simulink model "SMA_Model_with_Inverter_2021a"  (R2021a)
settings: Solver=ode45  StartTime=0.0  StopTime=300.0  FixedStep=1e-4  RelTol=1e-3
values from neighbouring files (symbols this model uses):
  a0 = 8.7e-7    (= 8.7e-07)    [Model_Parameters.m]
  a1 = 4.8e-8    (= 4.8e-08)    [Model_Parameters.m]
  a2 = -7.8e-9    (= -7.8e-09)    [Model_Parameters.m]
  a3 = 7e-10    [Model_Parameters.m]
  a4 = 3.7e-11    [Model_Parameters.m]
  c_heat = 837.36    [Model_Parameters.m]
  Capacitance = 10e-3    (= 0.01)    [Model_Parameters.m]
  CarrierFrequency = 1e-3    (= 0.001)    [Model_Parameters.m]
  Delta = 4.425e-2    (= 0.04425)    [Model_Parameters.m]
  do = 5e-4    (= 0.0005)    [Model_Parameters.m]
  Ea = 79    [Model_Parameters.m]
  Em = 34    [Model_Parameters.m]
  h = 70    [Model_Parameters.m]
  Initial_Rm = 1    [Model_Parameters.m]
  Initial_temperature = T_amb    (= 20)    [Model_Parameters.m]
  k = 58.19    [Model_Parameters.m]
  k1 = 0.0204    [Model_Parameters.m]
  k2 = 0.01293    [Model_Parameters.m]
  L = 0    [Model_Parameters.m]
  lo = 0.96    [Model_Parameters.m]
  m3 = 70    [Model_Parameters.m]
  mu_minus = 57    [Model_Parameters.m]
  mu_plus = 72    [Model_Parameters.m]
  n3 = 3    [Model_Parameters.m]
  ni_minus = 1    [Model_Parameters.m]
  ni_plus = 1    [Model_Parameters.m]
  p1 = 9.2e-7    (= 9.2e-07)    [Model_Parameters.m]
  p2 = 8.4e-7    (= 8.4e-07)    [Model_Parameters.m]
  p3 = 0.2499    [Model_Parameters.m]
  q1 = 3.4e-8    (= 3.4e-08)    [Model_Parameters.m]
  q2 = 5.7e-10    [Model_Parameters.m]
  R = 4.3    [Model_Parameters.m]
  rho = 6450    [Model_Parameters.m]
  sigma_minus = 1.6    [Model_Parameters.m]
  sigma_plus = 1.5    [Model_Parameters.m]
  Slider_Friction = 0.11    [Model_Parameters.m]
  SupplyInternalInductance = 0.4e-3    (= 0.0004)    [Model_Parameters.m]
  SupplyInternalResistance = 0.4    [Model_Parameters.m]
  SupplyVoltage = 80    [Model_Parameters.m]
  T_amb = 20    [Model_Parameters.m]
undefined symbols (not defined in the file or in its folder): CapacitanceResistance
libraries: fl_lib x7, spsVoltageMeasurementLib x6, spsDiodeLib x5, spsIdealSwitchLib x5, spsCurrentMeasurementLib x4, nesl_utility x4, spsSeriesRLCBranchLib x4, simulink x2, spsDCVoltageSourceLib x1, spspowerguiLib x1
settings Model: Creator=barag  LastModifiedBy=barag
settings SolverCC: ZeroCrossAlgorithm=Adaptive
settings DebuggingCC: MaskedZcDiagnostic=none  IgnoredZcDiagnostic=none

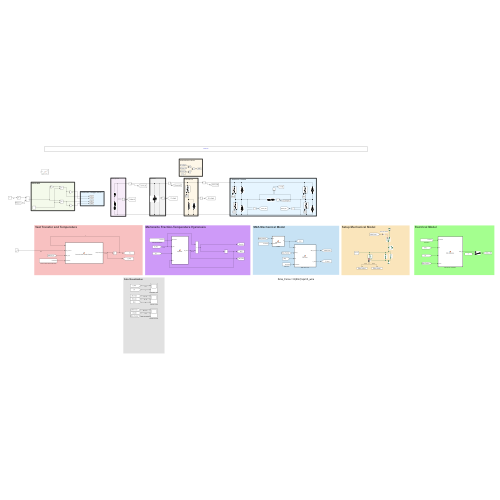
[thumbnail: Simulink's stored preview of the top-level diagram]
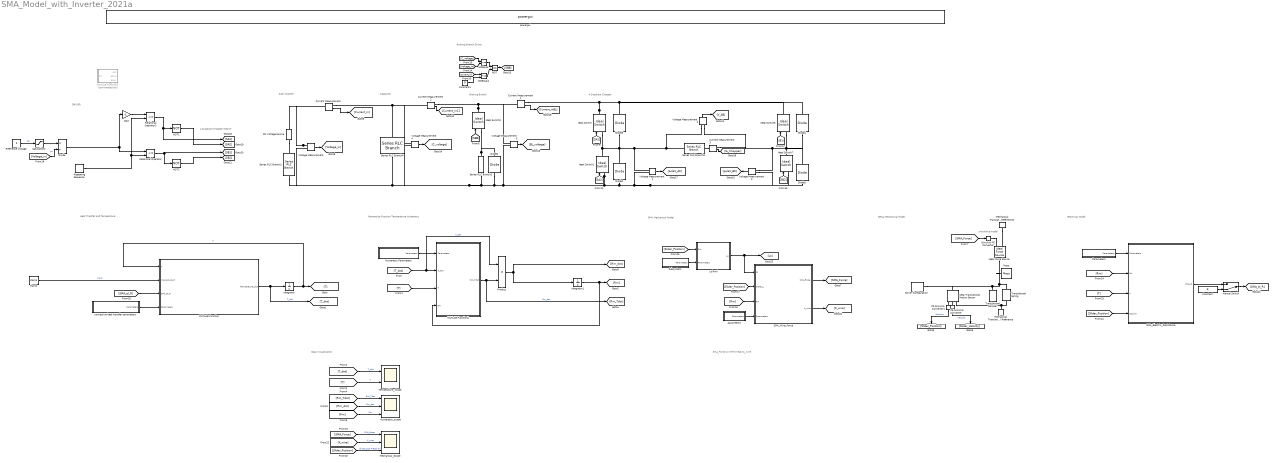
== system SMA_Model_with_Inverter_2021a ==
  note: Electrical Model
  note: Sma_Force = K(Rm)*eps*A_wire
  note: SMA Mechanical Model
  note: Setup Mechanical Model
  note: sma force model
  note: Data Visualization
  note: Martensite Fraction-Temperature Hysteresis
  note: Heat Transfer and Temperature
  note: Braking Branch
  note: Capacitor
  note: 4 Quadrant Chopper
  note: Braking Branch Driver
  note: Suply System
  note: DRIVER
  note: 4 Quadrant Chopper IN/OUT
  Constant : Constant  Value=R
  Constant1 : Constant  Value=0
  Current Measurement{,1..3} (4 alike) : spsCurrentMeasurementLib/Current Measurement  PhasorSimulation=off  OutputType=Complex  PSBequivalent=0
  DC Voltage Source : spsDCVoltageSourceLib/DC Voltage Source  Amplitude=SupplyVoltage  Measurements=None
  Diode{1..5} (5 alike) : spsDiodeLib/Diode  Ron=DiodeResistance  Lon=0  Vf=DiodeVfm  IC=0  UseSnubber=0  Rs=DiodeResistance  Cs=inf  Measurements=off
  Divide : Product  Inputs=*/
  Gain : Gain  Gain=-1
  Hysteresis Parameters : Subsystem
  Hysteresis_scope : Scope  NumInputPorts=3
  Ideal Force Source : fl_lib/Mechanical/Mechanical Sources/Ideal Force Source
  Ideal Switch{,1..2,6..7} (5 alike) : spsIdealSwitchLib/Ideal Switch  Ron=MosfetResistance  Lon=0  IC=0  Rs=DiodeResistance  Cs=inf  Measurements=off
  Ideal Translational Motion Sensor : fl_lib/Mechanical/Mechanical Sensors/Ideal Translational Motion Sensor  offset=4 cm
  Integrator : Integrator  InitialCondition=Initial_temperature
  Integrator1 : Integrator  InitialCondition=Initial_Rm
  Lo(Rm) : MATLAB Function  TreatAsAtomicUnit=on
  MATLAB Function : MATLAB Function  TreatAsAtomicUnit=on
  MATLAB Function1 : MATLAB Function  Commented=on  TreatAsAtomicUnit=on
  MATLAB Function2 : MATLAB Function  TreatAsAtomicUnit=on
  Manual Switch : ManualSwitch  CurrentSetting=0
  Mass : fl_lib/Mechanical/Translational Elements/Mass  mass=Slider_Mass kg  num_ports=foundation.enum.numPorts2.one  v_specify=off  v_priority=High  v=0 m/s  v_nominal_specify=off  v_nominal_unit=m/s  v_nominal_value=1  f_specify=off  f_priority=None  f=0 N  f_nominal_specify=off  f_nominal_unit=N  f_nominal_value=1
  Mechanical Translational Reference : fl_lib/Mechanical/Translational Elements/Mechanical Translational Reference
  Mechanical Translational Reference1 : fl_lib/Mechanical/Translational Elements/Mechanical Translational Reference
  Mechanical_Scope : Scope  NumInputPorts=3
  NOT : Logic  IconShape=distinctive  AllPortsSameDT=off  OutDataTypeStr=boolean
  NOT1 : Logic  Operator=NOT  IconShape=distinctive  AllPortsSameDT=off  OutDataTypeStr=boolean
  NOT2 : Logic  Operator=NOT  IconShape=distinctive  AllPortsSameDT=off  OutDataTypeStr=boolean
  NotEqual : RelationalOperator  Operator=~=  OutDataTypeStr=boolean  RndMeth=Simplest
  NotEqual1 : RelationalOperator  Operator=<=  OutDataTypeStr=boolean  RndMeth=Simplest
  PS-Simulink Converter : nesl_utility/PS-Simulink Converter  PhysicalDomain=network_engine_domain  SubClassName=ps_output  LeftPortType=input  RightPortType=output  PseudoPeriodic=off  Frequencies=[]  Unit=inherit  AffineConversion=off
      settings: SourceProductBaseCode=PW,SS
  PS-Simulink Converter1 : nesl_utility/PS-Simulink Converter  PhysicalDomain=network_engine_domain  SubClassName=ps_output  LeftPortType=input  RightPortType=output  PseudoPeriodic=off  Frequencies=[]  Unit=inherit  AffineConversion=off
      settings: SourceProductBaseCode=PW,SS
  Parameters : Subsystem
  Product : Product
  Ramp : simulink/Sources/Ramp  slope=0.3  start=0  InitialOutput=0
  Reference Voltage : Constant
  Relational Operator : RelationalOperator  Operator=<=  OutDataTypeStr=boolean  RndMeth=Simplest
  Relational Operator1 : RelationalOperator  Operator=<=  OutDataTypeStr=boolean  RndMeth=Simplest
  Repeating Sequence : simulink/Sources/Repeating Sequence  rep_seq_t=[0 (CarrierFrequency)/2 CarrierFrequency]  rep_seq_y=[-1 1 -1]
  SMA_Electric_Resistance : MATLAB Function  TreatAsAtomicUnit=on
  SMA_Wire_Force : MATLAB Function  TreatAsAtomicUnit=on
  Saturation2 : Saturate  UpperLimit=79.94  LowerLimit=-79.94
  Series RLC Branch1 : spsSeriesRLCBranchLib/Series RLC Branch  LConnTagsString=__new0  RConnTagsString=__new0  BranchType=RL  Resistance=SupplyInternalResistance  Inductance=SupplyInternalInductance  SetiL0=off  InitialCurrent=0  Capacitance=1  Setx0=off  InitialVoltage=0  Measurements=None
  Series RLC Branch2 : spsSeriesRLCBranchLib/Series RLC Branch  LConnTagsString=__new0  RConnTagsString=__new0  BranchType=R  Resistance=10  Inductance=10e-3  SetiL0=off  InitialCurrent=0  Capacitance=1  Setx0=off  InitialVoltage=0  Measurements=None
  Series RLC Branch3 : spsSeriesRLCBranchLib/Series RLC Branch  LConnTagsString=__new0  RConnTagsString=__new0  BranchType=RL  Resistance=R  Inductance=L  SetiL0=off  InitialCurrent=0  Capacitance=1  Setx0=off  InitialVoltage=0  Measurements=None
  Series RLC Branch4 : spsSeriesRLCBranchLib/Series RLC Branch  LConnTagsString=__new0  RConnTagsString=__new0  BranchType=C  Resistance=CapacitanceResistance  Inductance=10e-3  SetiL0=off  InitialCurrent=0  Capacitance=Capacitance  Setx0=on  InitialVoltage=0  Measurements=None
  Simulink-PS Converter : nesl_utility/Simulink-PS Converter  PhysicalDomain=network_engine_domain  SubClassName=ps_input  LeftPortType=input  RightPortType=output  PseudoPeriodic=off  Frequencies=[]  NoiseDistribution=none  NoiseParameters=[]  Unit=1  AffineConversion=off  FilteringAndDerivatives=provide  SimscapeFilterOrder=1  InputFilterTimeConstant=0.001  UdotUserProvided=0
      settings: SourceProductBaseCode=PW,SS
  Solver Configuration : nesl_utility/Solver Configuration  PhysicalDomain=network_engine_domain  SubClassName=solver  LeftPortType=input  RightPortType=generic  Tones=[]  Harmonics=[]  SimulateNoise=off  Profile=off  UseLocalSampling=off  EnableSwitchedLinearOptims=on  FrequencyDomain=off  UseCCode=off  RelTol=0.001  AbsTol=1e-06  MinStep=1e-09  ToWorkspace=off  RevertToSquareIcSolve=off  NumHomotopyIterations=100  PhasorMode=off  PhasorModeNumHarmonics=1  DoDC=off  ResidualTolerance=1e-09  UseLocalSolver=off  LocalSolverChoice=NE_BACKWARD_EULER_ADVANCER  LocalSolverSampleTime=0.001  DoFixedCost=off  MaxNonlinIter=3  MaxModeIter=2  ComputeImpulses=off  ImpulseIterations=2  LinearAlgebra=auto  EquationFormulation=NE_TIME_EF  DelaysMemoryBudget=1024  AutomaticFiltering=on  FilteringTimeConstant=0.001  PartitionStorageMethod=AS_NEEDED  PartitionMemoryBudget=1024  PartitionMethod=ROBUST
      settings: SourceProductBaseCode=PW,SS
  Subsystem : Subsystem
  Temperature_scope : Scope  NumInputPorts=2
  Translational Damper : fl_lib/Mechanical/Translational Elements/Translational Damper  D=Slider_Friction N/(m/s)  v_specify=off  v_priority=None  v=0 m/s  v_nominal_specify=off  v_nominal_unit=m/s  v_nominal_value=1  f_specify=off  f_priority=None  f=0 N  f_nominal_specify=off  f_nominal_unit=N  f_nominal_value=1
  Translational Spring : fl_lib/Mechanical/Translational Elements/Translational Spring  spr_rate=Spring_Stiff N/m  v_specify=off  v_priority=None  v=0 m/s  v_nominal_specify=off  v_nominal_unit=m/s  v_nominal_value=1  f_specify=off  f_priority=High  f=9 N  f_nominal_specify=off  f_nominal_unit=N  f_nominal_value=1  x_specify=off  x_priority=High  x=0 m  x_nominal_specify=off  x_nominal_unit=m  x_nominal_value=1
  Voltage Measurement{,1..5} (6 alike) : spsVoltageMeasurementLib/Voltage Measurement  PhasorSimulation=off  OutputType=Complex  PSBequivalent=0
  convective heat transfer parameters : Subsystem
  parameters : Subsystem
  powergui : spspowerguiLib/powergui  Priority=1  SimulationMode=Continuous  SampleTime=50e-6  frequency=60  Iterations=50  frequencyindice=0  Pbase=100e6  ErrMax=1e-4  UnitsV=kV  UnitsW=MW  buscounter=0  FunctionMessages=off  echomessages=off  EnableUseOfTLC=off  CurrentSourceSwitches=off  DisableSnubberDevices=off  DisableRonSwitches=off  DisableVfSwitches=off  DisplayEquations=off  AutomaticDiscreteSolvers=off  SolverType=Tustin/Backward Euler (TBE)  Interpol=off  ExternalGateDelay=off  methode=off  Ts=100  x0status=blocks  SPID=on  SwTol=0  HookPort=off  NonlinearTolerance=1e-4  nMaxIteration=100  ContinueOnMaxIteration=off  RestoreLinks=warning  ResistiveCurrentMeasurement=off  Frange=[0:2:500]  Ylog=off  Xlog=on  ShowGrid=off  save=off  variable=ZData  structure=0  ZoomFFT=off  StartTime=0.0  cycles=1  DisplayStyle=1  fundamental=60  FreqAxis=off  MaxFrequency=1000  frequencyindicesteady=1  RmsSteady=1  display=off
  wires:
  MATLAB Function/1(Temperature_dot) -> [T_dot], Integrator/1  "T_dot"
  Integrator/1 -> MATLAB Function/1(T), [T]  "T"
  convective heat transfer parameters/1(Parameters) -> MATLAB Function/4(Parameters)
  Hysteresis Parameters/1(Parameters) -> MATLAB Function2/1(Parameters)
  [T_dot] -> MATLAB Function2/2(T_dot), Product/1  "T_dot"
  MATLAB Function2/1(Rm_Tdot) -> Product/2, [Rm_Tdot]  "Rm_dot"
  [T_dot] -> Temperature_scope/1  "T_dot"
  [T] -> Temperature_scope/2  "T"
  [Rm_Tdot] -> Hysteresis_scope/1  "Rm_Tdot"
  [Rm_dot] -> Hysteresis_scope/2  "Rm_dot"
  [Rm] -> Hysteresis_scope/3  "Rm"
  Integrator1/1 -> [Rm], MATLAB Function2/4(Rm)
  [T] -> MATLAB Function2/3(T)
  PS-Simulink Converter/1 -> [Slider_Velocity]  "Velocity"
  PS-Simulink Converter1/1 -> [Slider_Position]  "Position"
  [SMA_Force] -> Simulink-PS Converter/1
  Voltage Measurement2/1 -> [V_AB]
  Voltage Measurement3/1 -> [poleV_B0]
  Current Measurement1/1 -> [Current_inBL]
  [SB1] -> Ideal Switch6/1
  [C_voltage] -> NotEqual/1
  Current Measurement/1 -> [Current_in]
  NotEqual/1 -> NOT/1
  Voltage Measurement1/1 -> [poleV_A0]
  [SA2] -> Ideal Switch1/1
  Voltage Measurement/1 -> [Voltage_in]
  [Current_in] -> NotEqual1/1
  Current Measurement2/1 -> [Current_inC]
  [SBB] -> Ideal Switch2/1
  Constant1/1 -> NotEqual1/2
  [SB2] -> Ideal Switch7/1
  NotEqual1/1 -> NOT/2
  NOT/1 -> [SBB]
  Voltage Measurement4/1 -> [C_voltage]
  Voltage Measurement5/1 -> [BL_voltage]
  [SA1] -> Ideal Switch/1
  Current Measurement3/1 -> [Ia_Chopper]
  [Voltage_in] -> NotEqual/2
  Divide/1 -> Relational Operator/1, Gain/1
  Repeating Sequence/1 -> Relational Operator1/2, Relational Operator/2
  Gain/1 -> Relational Operator1/1
  NOT2/1 -> [SB2]
  Relational Operator1/1 -> [SA1], NOT1/1
  NOT1/1 -> [SA2]
  Relational Operator/1 -> [SB1], NOT2/1
  Saturation2/1 -> Divide/1
  Reference Voltage/1 -> Saturation2/1  "Va*"
  [Voltage_in] -> Divide/2  "Vin"
  parameters/1(Parameters) -> SMA_Wire_Force/4(Parameters)
  [Rm] -> SMA_Wire_Force/3(Rm)
  SMA_Wire_Force/1(SMA_Force) -> [SMA_Force]
  [Slider_Position] -> SMA_Wire_Force/2(Delta_L)
  [SMA_Force] -> Mechanical_Scope/1  "SMA_force"
  [Slider_Position] -> Mechanical_Scope/3  "Slider_pos = Espilon"
  SMA_Wire_Force/2(K_wire) -> [K_wire]
  [K_wire] -> Mechanical_Scope/2  "K_wire"
  [Slider_Position] -> SMA_Electric_Resistance/4(epsilon)
  [T] -> SMA_Electric_Resistance/3(T)
  [Rm] -> SMA_Electric_Resistance/2(Rm)
  Parameters/1(Parameters) -> SMA_Electric_Resistance/1(Parameters)
  Subsystem/1(Parameters) -> Lo(Rm)/2(Parameters)
  [Slider_Position] -> Lo(Rm)/1(Rm)
  Lo(Rm)/1(Lo) -> [Lo], SMA_Wire_Force/1(Lo)
  SMA_Electric_Resistance/1(SMA_R) -> Manual Switch/1
  Ramp/1 -> MATLAB Function/2(Input_Current)  "Input"
  [SMA_el_R] -> MATLAB Function/3(SMA_el_R)
  Product/1 -> Integrator1/1, [Rm_dot]
  Manual Switch/1 -> [SMA_el_R]
  Constant/1 -> Manual Switch/2
  connections:
  Translational Damper/RConn1 -- Ideal Translational Motion Sensor/RConn1 -- Translational Spring/RConn1 -- Mechanical Translational Reference/LConn1
  Translational Damper/LConn1 -- Solver Configuration/RConn1 -- Ideal Translational Motion Sensor/LConn1 -- Mass/LConn1 -- Ideal Force Source/LConn1 -- Translational Spring/LConn1
  Mechanical Translational Reference1/LConn1 -- Ideal Force Source/RConn2
  PS-Simulink Converter/LConn1 -- Ideal Translational Motion Sensor/RConn2
  PS-Simulink Converter1/LConn1 -- Ideal Translational Motion Sensor/RConn3
  Simulink-PS Converter/RConn1 -- Ideal Force Source/RConn1
  Voltage Measurement/LConn1 -- DC Voltage Source/RConn1 -- Current Measurement/LConn1
  Voltage Measurement3/LConn1 -- Voltage Measurement2/LConn2 -- Current Measurement3/RConn1 -- Ideal Switch6/LConn1 -- Diode4/LConn1 -- Diode5/RConn1 -- Ideal Switch7/RConn1
  Series RLC Branch2/LConn1 -- Ideal Switch2/LConn1 -- Diode2/RConn1
  Ideal Switch1/LConn1 -- Voltage Measurement5/LConn2 -- Voltage Measurement4/LConn2 -- Voltage Measurement/LConn2 -- Series RLC Branch1/RConn1 -- Series RLC Branch4/RConn1 -- Series RLC Branch2/RConn1 -- Diode2/LConn1 -- Diode1/LConn1 -- Voltage Measurement3/LConn2 -- Ideal Switch7/LConn1 -- Diode5/LConn1 -- Voltage Measurement1/LConn2
  Ideal Switch2/RConn1 -- Current Measurement2/RConn1 -- Current Measurement1/LConn1 -- Voltage Measurement5/LConn1
  Series RLC Branch4/LConn1 -- Voltage Measurement4/LConn1 -- Current Measurement2/LConn1 -- Current Measurement/RConn1
  Series RLC Branch3/LConn1 -- Voltage Measurement1/LConn1 -- Ideal Switch/LConn1 -- Ideal Switch1/RConn1 -- Diode1/RConn1 -- Diode3/LConn1 -- Voltage Measurement2/LConn1
  Ideal Switch/RConn1 -- Current Measurement1/RConn1 -- Diode3/RConn1 -- Ideal Switch6/RConn1 -- Diode4/RConn1
  DC Voltage Source/LConn1 -- Series RLC Branch1/LConn1
  Series RLC Branch3/RConn1 -- Current Measurement3/LConn1

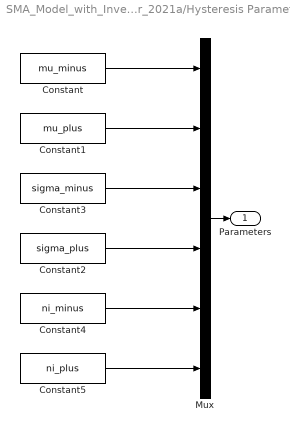
== system SMA_Model_with_Inverter_2021a/Hysteresis Parameters ==
  Constant : Constant  Value=mu_minus
  Constant1 : Constant  Value=mu_plus
  Constant2 : Constant  Value=sigma_plus
  Constant3 : Constant  Value=sigma_minus
  Constant4 : Constant  Value=ni_minus
  Constant5 : Constant  Value=ni_plus
  Mux : Mux  Inputs=6
  Parameters : Outport
  wires:
  Mux/1 -> Parameters/1
  Constant2/1 -> Mux/4
  Constant/1 -> Mux/1
  Constant4/1 -> Mux/5
  Constant1/1 -> Mux/2
  Constant5/1 -> Mux/6
  Constant3/1 -> Mux/3

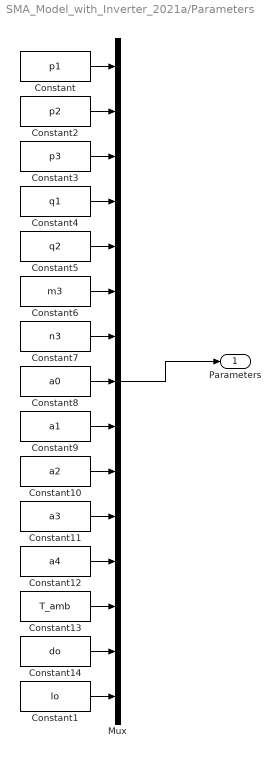
== system SMA_Model_with_Inverter_2021a/Parameters ==
  Constant : Constant  Value=p1
  Constant1 : Constant  Value=lo
  Constant10 : Constant  Value=a2
  Constant11 : Constant  Value=a3
  Constant12 : Constant  Value=a4
  Constant13 : Constant  Value=T_amb
  Constant14 : Constant  Value=do
  Constant2 : Constant  Value=p2
  Constant3 : Constant  Value=p3
  Constant4 : Constant  Value=q1
  Constant5 : Constant  Value=q2
  Constant6 : Constant  Value=m3
  Constant7 : Constant  Value=n3
  Constant8 : Constant  Value=a0
  Constant9 : Constant  Value=a1
  Mux : Mux  Inputs=15
  Parameters : Outport
  wires:
  Constant10/1 -> Mux/10
  Constant3/1 -> Mux/3
  Constant12/1 -> Mux/12
  Constant2/1 -> Mux/2
  Constant8/1 -> Mux/8
  Constant4/1 -> Mux/4
  Constant7/1 -> Mux/7
  Constant/1 -> Mux/1
  Constant5/1 -> Mux/5
  Constant11/1 -> Mux/11
  Constant13/1 -> Mux/13
  Constant14/1 -> Mux/14
  Constant6/1 -> Mux/6
  Constant9/1 -> Mux/9
  Mux/1 -> Parameters/1
  Constant1/1 -> Mux/15

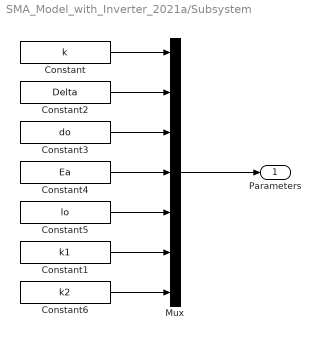
== system SMA_Model_with_Inverter_2021a/Subsystem ==
  Constant : Constant  Value=k
  Constant1 : Constant  Value=k1
  Constant2 : Constant  Value=Delta
  Constant3 : Constant  Value=do
  Constant4 : Constant  Value=Ea
  Constant5 : Constant  Value=lo
  Constant6 : Constant  Value=k2
  Mux : Mux  Inputs=7
  Parameters : Outport
  wires:
  Constant/1 -> Mux/1
  Mux/1 -> Parameters/1
  Constant4/1 -> Mux/4
  Constant2/1 -> Mux/2
  Constant3/1 -> Mux/3
  Constant5/1 -> Mux/5
  Constant1/1 -> Mux/6
  Constant6/1 -> Mux/7

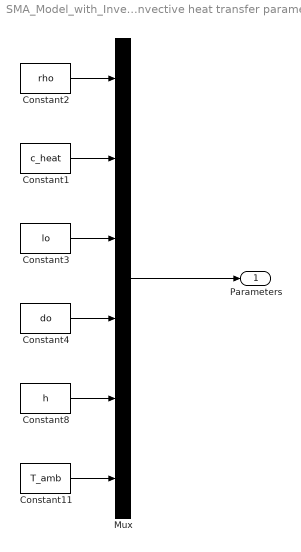
== system SMA_Model_with_Inverter_2021a/convective heat transfer parameters ==
  Constant1 : Constant  Value=c_heat
  Constant11 : Constant  Value=T_amb
  Constant2 : Constant  Value=rho
  Constant3 : Constant  Value=lo
  Constant4 : Constant  Value=do
  Constant8 : Constant  Value=h
  Mux : Mux  Inputs=6
  Parameters : Outport
  wires:
  Constant8/1 -> Mux/5
  Constant2/1 -> Mux/1
  Constant1/1 -> Mux/2
  Constant3/1 -> Mux/3
  Constant4/1 -> Mux/4
  Mux/1 -> Parameters/1
  Constant11/1 -> Mux/6

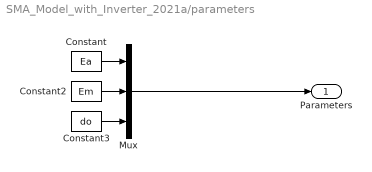
== system SMA_Model_with_Inverter_2021a/parameters ==
  Constant : Constant  Value=Ea
  Constant2 : Constant  Value=Em
  Constant3 : Constant  Value=do
  Mux : Mux  Inputs=3
  Parameters : Outport
  wires:
  Constant2/1 -> Mux/2
  Constant3/1 -> Mux/3
  Constant/1 -> Mux/1
  Mux/1 -> Parameters/1

== matlab function SMA_Model_with_Inverter_2021a/MATLAB Function1 ==
  data: Rm input; eps output; eps_o output; eps_r output
function [eps,eps_o,eps_r]= Epsilon(Rm)

c1 = pi*(do^2)*(Ea + (Em - Ea)*Rm);
d1 = -4*k*Lo - c1*(1-(2*eps_o));
e1 = 4*k*Delta - c1*eps_o*(1-eps_o);

c2 = pi*(do^2)*(Ea + (ET - Ea)*Rm);
d2 = -4*k*Lo -c2*(1-(2*eps_o)) +  pi*(do^2)*Rm*eps_ym*(Em - ET);
e2 = 4*k*Delta -c2*eps_o*(1-eps_o) + Rm*eps_ym*(Em - ET);

c3 = pi*(do^2)*(Ea + (Ed - Ea)*Rm);
d3 = -4*k*Lo -c3*(1-(2*eps_o)) + pi*(do^2)*Rm*(eps_ym*(Em - ET) + eps_dm*(ET - Ed));
e3 = 4*k*Delta -c3*eps_o*(1-eps_o) + Rm*(eps_ym*(Em - ET) + eps_dm*(ET - Ed));



Epsilon = 0;

== matlab function SMA_Model_with_Inverter_2021a/MATLAB Function ==
  data: T input; Input_Current input; SMA_el_R input; Parameters input; Temperature_dot output
function Temperature_dot = Convective_Heat_Transfer_Equation( T, Input_Current, SMA_el_R, Parameters)
% Parameters Estraztion
rho =    Parameters(1); % mass density of SMA wire[kgm-3]
c_heat = Parameters(2); % specific heat of SMA wire [Jkg-1C-1]
lo =     Parameters(3); % undeformed SMA wire length in 100% A state [m]
do =     Parameters(4); % cross-sectional diameter of undeformed SMA wire [m]
h =      Parameters(5); % convection heat transfer coefficient [Wm-2C-1]
T_amb =  Parameters(6); % ambient temperature [C]

% Equation Terms Definitions:
Term_1 = (rho*c_heat*pi*lo*(do^2))/4;
%Term_2 = (1+(eps/2))*p1*do*Lo*h;
Term_2_simplified = pi*do*lo*h;
El_Pow_Term = SMA_el_R*(Input_Current^2);
T_diff = T - T_amb;

% Temperature Rate of Variation :
Temperature_dot = (El_Pow_Term - Term_2_simplified*T_diff)/Term_1; %
%Simplified version with eps assumed to be small and neglectable
%Temperature_dot = (El_Pow_Term - Term_2*T_diff)/Term_1;

== matlab function SMA_Model_with_Inverter_2021a/MATLAB Function2 ==
  data: Parameters input; Rm_Tdot output; T_dot input; T input; Rm input
function Rm_Tdot = Hysteresis(Parameters, T_dot, T, Rm)
    % Parameter Extraction
    mu_minus =    Parameters(1);
    mu_plus =     Parameters(2);
    sigma_minus = Parameters(3);
    sigma_plus =  Parameters(4);
    ni_minus =    Parameters(5);
    ni_plus =     Parameters(6);

    ER_minus = erf((T-mu_minus)/(sigma_minus*sqrt(2)));
    ER_plus = erf((T-mu_plus)/(sigma_plus*sqrt(2)));

    H_minus = 0.5 * (1 + ER_minus);
    H_plus  = 0.5 * (1 + ER_plus);

    Exp_minus = exp(-((T-mu_minus)/(sigma_minus*sqrt(2)))^2);
    Exp_plus  = exp(-((T-mu_plus)/(sigma_plus*sqrt(2)))^2);

    Gauss_minus= (1/(sigma_minus*sqrt(2*pi)))*Exp_minus;
    Gauss_plus = (1/(sigma_plus*sqrt(2*pi)))*Exp_plus;
    
    Rm_Tdot=0;
    if T_dot >= 0
        ceff_plus = (H_minus + Rm - 1)/(H_plus - H_minus + 0.0000001);
        Rm_Tdot = ceff_plus*Gauss_plus*ni_plus;
    elseif T_dot < 0
        ceff_minus = (H_plus + Rm - 1)/(H_minus - H_plus +0.001);
        Rm_Tdot = ceff_minus*Gauss_minus*ni_minus;
    end 
%   if Rm_Tdot == 0
%       Rm_Tdot = 1e-6;
%   end
end

== matlab function SMA_Model_with_Inverter_2021a/SMA_Wire_Force ==
  data: Lo input; Delta_L input; SMA_Force output; Rm input; Parameters input; K_wire output
function [SMA_Force, K_wire]= SMA_force(Lo, Delta_L, Rm, Parameters)
% Parameters
Ea = Parameters(1);
Em = Parameters(2);
do = Parameters(3);

% Wire sectional area
A_wire = (do/2)^2 * pi;

% Wire Stiffness Coefficient
K_wire = Rm*Em + (1-Rm)*Ea;

% deformation
epsilon = Delta_L/Lo;

% Force generated by the SMA wire 
SMA_Force = K_wire * epsilon * A_wire;

== matlab function SMA_Model_with_Inverter_2021a/SMA_Electric_Resistance ==
  data: Parameters input; SMA_R output; Rm input; T input; epsilon input
function SMA_R = SMA_Resistance(Parameters, Rm, T, epsilon)
% Initialization
SMA_R = 0;

% Parameters Extraction
p1 = Parameters(1); % [Ohm*m] 
p2 = Parameters(2); % [Ohm*m] 
p3 = Parameters(3); % [C-1]
q1 = Parameters(4); % [Ohm*m] 
q2 = Parameters(5); % [Ohm*m / C]
m3 = Parameters(6); % [C]
n3 = Parameters(7); % [C]
a0 = Parameters(8); % [Ohm*m]
a1 = Parameters(9); % [Ohm*m / C]
a2 = Parameters(10);% [Ohm*m / C2]
a3 = Parameters(11);% [Ohm*m / C3]
a4 = Parameters(12);% [Ohm*m / C4]
T_amb = Parameters(13); %[C]
do = Parameters(14); % [m]
lo = Parameters(15); % [m]

% Wire sectional area
A_wire = (do/2)^2 * pi;

% Resistivity
rho_a = p1 + p2*exp(-p3*(T-T_amb));
rho_m = (q1-q2*T)*(1 + erf((T-m3)/n3)) + a0 + a1*(T-T_amb) + a2*(T-T_amb)^2 + a3*(T-T_amb)^3 + a4*(T-T_amb)^4;

% Conductivity
GG = (A_wire/(lo*(1+2*epsilon)))*((1-Rm)/rho_a + Rm/rho_m);

%SMA Wire Electical Resistance
SMA_R = 1/GG;

== matlab function SMA_Model_with_Inverter_2021a/Lo(Rm) ==
  data: Rm input; Lo output; Parameters input
function Lo = Initial_lenght(Rm, Parameters)

% Parameters
k     = Parameters(1);
Delta = Parameters(2);
do    = Parameters(3);
Ea    = Parameters(4)*(10^3);
lo    = Parameters(5);
k1    = Parameters(5);
k2    = Parameters(5);


% Wire sectional area
%A_wire = (do/2)^2 * pi;

%eps_0 = (1 - sqrt(1 - (4*k*Delta)/(A_wire*Ea)))/2;
eps_0 = 0;

eps_r = k1*Rm + k2*(Rm^2);

Lo = ( 1 + eps_0 + eps_r ) * lo;
